simulink model "EnabledGenerator1_Model"  (R2025a)
settings: Solver=VariableStepAuto  StartTime=0.0  StopTime=10.0  RelTol=1e-3
libraries: NSA_DEVS_SOURCES x2, NSA_DEVS_SINKS x2, NSA_DEVS_LOGISTICS x1
settings Model: Creator=david  LastModifiedBy=peter
settings RTWCC: GPUComputeCapability=3.5

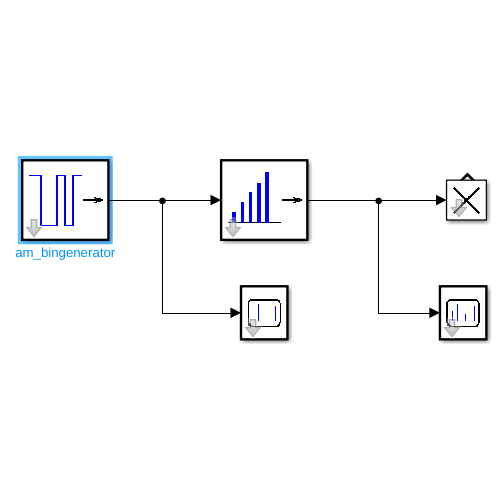
[thumbnail: Simulink's stored preview of the top-level diagram]
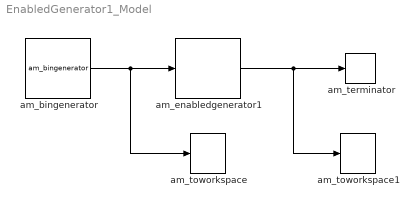
== system EnabledGenerator1_Model ==
  am_bingenerator : NSA_DEVS_SOURCES/am_bingenerator  z0=true  tVec=[2.4, 2.5, 2.7, 3.2, 100]  tau=[0,1]  debug=0
      settings: SourceProductName=Sources
  am_enabledgenerator1 : NSA_DEVS_SOURCES/am_enabledgenerator  tG=1  n0=1  nG=4  tD=[0,2]  tau=[0,1]  debug=0
      settings: SourceProductName=Sources
  am_terminator : NSA_DEVS_LOGISTICS/am_terminator  tau=[0,1]  debug=0
      settings: SourceProductName=Logistics
  am_toworkspace : NSA_DEVS_SINKS/am_toworkspace  varname="\"bingenOut\""  t0=0  format="\"vector\""  tau=[0,3]  debug=0
      settings: SourceProductName=Sinks
  am_toworkspace1 : NSA_DEVS_SINKS/am_toworkspace  varname="\"genOut\""  t0=0  format="\"vector\""  tau=[0,3]  debug=0
      settings: SourceProductName=Sinks
  wires:
  am_bingenerator/1 -> am_enabledgenerator1/1, am_toworkspace/1
  am_enabledgenerator1/1 -> am_toworkspace1/1, am_terminator/1
